simulink model "Newton_Rhapson"  (R2020b)
settings: Solver=VariableStepAuto  StartTime=0.0  StopTime=10.0  RelTol=1e-3
settings Model: Creator=Luke  LastModifiedBy=Luke

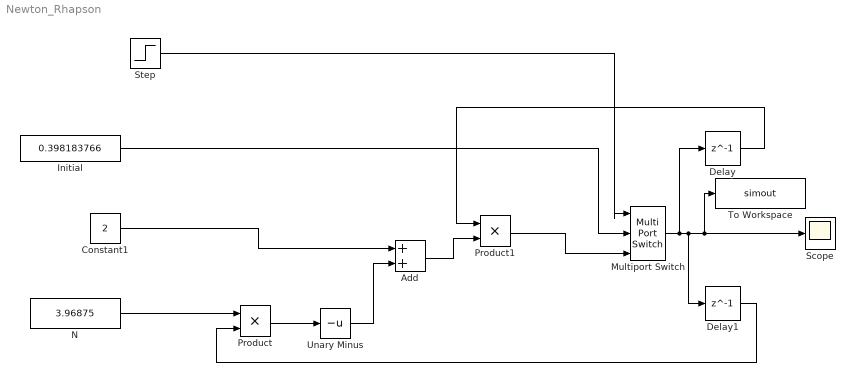
== system Newton_Rhapson ==
  Add : Sum
  Constant1 : Constant  Value=2
  Delay : Delay  DelayLength=1  InitialCondition=0
  Delay1 : Delay  DelayLength=1  InitialCondition=0
  Initial : Constant  Value=0.398183766
  Multiport Switch : MultiPortSwitch  DataPortOrder=Zero-based contiguous  Inputs=2  zeroidx=on
  N : Constant  Value=3.96875
  Product : Product
  Product1 : Product
  Scope : Scope
  Step : Step  SampleTime=0
  To Workspace : ToWorkspace  VariableName=simout  SaveFormat=Timeseries  SampleTime=-1
  Unary Minus : UnaryMinus
  wires:
  Multiport Switch/1 -> Delay/1, Delay1/1, To Workspace/1, Scope/1
  N/1 -> Product/1
  Add/1 -> Product1/2
  Product/1 -> Unary Minus/1
  Unary Minus/1 -> Add/2
  Constant1/1 -> Add/1
  Product1/1 -> Multiport Switch/3
  Initial/1 -> Multiport Switch/2
  Step/1 -> Multiport Switch/1
  Delay1/1 -> Product/2
  Delay/1 -> Product1/1
